simulink model "f_c"  (R2013a)
settings: Solver=ode45  StartTime=0.0  StopTime=10.0  RelTol=1e-3
settings Model: Creator=root  LastModifiedBy=root

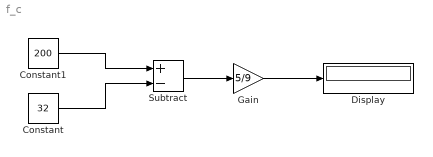
== system f_c ==
  Constant : Constant  Value=32
  Constant1 : Constant  Value=200
  Display : Display
  Gain : Gain  Gain=5/9
  Subtract : Sum  Inputs=+-
  wires:
  Constant/1 -> Subtract/2
  Gain/1 -> Display/1
  Constant1/1 -> Subtract/1
  Subtract/1 -> Gain/1
